simulink model "Actuator_Control"  (R2014a)
settings: Solver=FixedStepDiscrete  StartTime=0.0  StopTime=inf  FixedStep=sample_time  RelTol=1e-3
values from neighbouring files (symbols this model uses):
  A1_notch_f1 = -2*cos(fnotch_f1*sample_time)    [actuator_control_params.m]
  A2_notch_f1 = 1    [actuator_control_params.m]
  A_lpf_accel = 1 + B1_lpf_accel + B2_lpf_accel    [actuator_control_params.m]
  A_lpf_dtau = 1 + B1_lpf_dtau + B2_lpf_dtau    [actuator_control_params.m]
  B1_lpf_accel = -2*exp(-lpf_damping*fcut_acceleration*sample_time)*cos(fcut_acceleration*sample_time*sqrt(1-lpf_damping^2))    [actuator_control_params.m]
  B1_lpf_dtau = -2*exp(-lpf_damping*fcut_dtau*sample_time)*cos(fcut_dtau*sample_time*sqrt(1-lpf_damping^2))    [actuator_control_params.m]
  B1_notch_f1 = -2*exp(-notch_damping*fnotch_f1*sample_time)*cos(fnotch_f1*sample_time*sqrt(1-notch_damping^2))    [actuator_control_params.m]
  B2_lpf_accel = exp(-2*lpf_damping*fcut_acceleration*sample_time)    [actuator_control_params.m]
  B2_lpf_dtau = exp(-2*lpf_damping*fcut_dtau*sample_time)    [actuator_control_params.m]
  B2_notch_f1 = exp(-2*notch_damping*fnotch_f1*sample_time)    [actuator_control_params.m]
  j_segments = [0.145 0.155 0.145 0.155]    [model_params.m]
  k_ff = 1    [actuator_control_params.m]
  K_notch_f1 = (1+B1_notch_f1+B2_notch_f1)/(1+A1_notch_f1+A2_notch_f1)    [actuator_control_params.m]
  k_sea = [4255.0 4525.3 4372.1 4322.4]    [model_params.m]
  kd_sea_torque_flight = 0.3*sqrt(2)/2*2*sqrt(k_sea.*j_segments) ./ k_sea    [actuator_control_params.m]
  kd_sea_torque_stance = sqrt(2)/2*2*sqrt(k_sea.*(4.4)) ./ k_sea    [actuator_control_params.m]
  kp_sea_torque_flight = 0.3    [actuator_control_params.m]
  kp_sea_torque_stance = 8    [actuator_control_params.m]
  lateral_torque_ramp_time = control_start_time+2    (= 11)    [actuator_control_params.m]
  max_sagittal_loaded_torque = LEG_MTR_MAX_TORQUE    [actuator_control_params.m]
  max_sagittal_unloaded_torque = LEG_MTR_MAX_CONT_TORQUE    [actuator_control_params.m]
  sagittal_torque_ramp_time = sagittal_starting_time+5    (= 18)    [actuator_control_params.m]
  sea_control_torque_cmd_small_threshold = 1*ones(1,4)    [actuator_control_params.m]
  sea_coulomb_friction = [18.69 26.08 25.95 26.8+5]    [actuator_control_params.m]
  sea_coulomb_friction_direction_switch_sensitivity = [15 5 15 15]    [actuator_control_params.m]
  sea_extra_sliding_friction = 0.001*ones(1,4)    [actuator_control_params.m]
  sea_offset_friction = [7.659 -6.198 6.447 -6.594]    [actuator_control_params.m]
  stance_flight_torque_threshold = 40*ones(1,4)    [actuator_control_params.m]
undefined symbols (not defined in the file or in its folder): sample_time
libraries: simulink x7
settings Model: BufferReuse=off  Creator=wmartin  LastModifiedBy=wmartin
settings SolverCC: EnableConcurrentExecution=on
settings DataIOCC: SaveOutput=off  SaveTime=off
settings OptimizationCC: BlockReduction=off  OptimizeBlockIOStorage=off  BufferReuse=off  GlobalBufferReuse=off  ExpressionFolding=off  LocalBlockOutputs=off  SimCompilerOptimization=On
settings HardwareCC: ProdIntDivRoundTo=Zero  ProdEndianess=LittleEndian  ProdHWDeviceType=Generic->32-bit x86 compatible
settings ModelReferenceCC: ModelReferenceNumInstancesAllowed=Single  ModelReferenceMinAlgLoopOccurrences=on
settings RTWCC: SystemTargetFile=slrt.tlc  TemplateMakefile=slrt_default_tmf  Description=Simulink Real-Time  RTWVerbose=off  ProcessScript=slrt_make_rtw_hook  RTWCompilerOptimization=On
settings SimulinkRealTimeCC: GeneratePreprocessorConditionals=Disable all  EnableShiftOperators=on  RL32LogBufSizeModifier=100000000

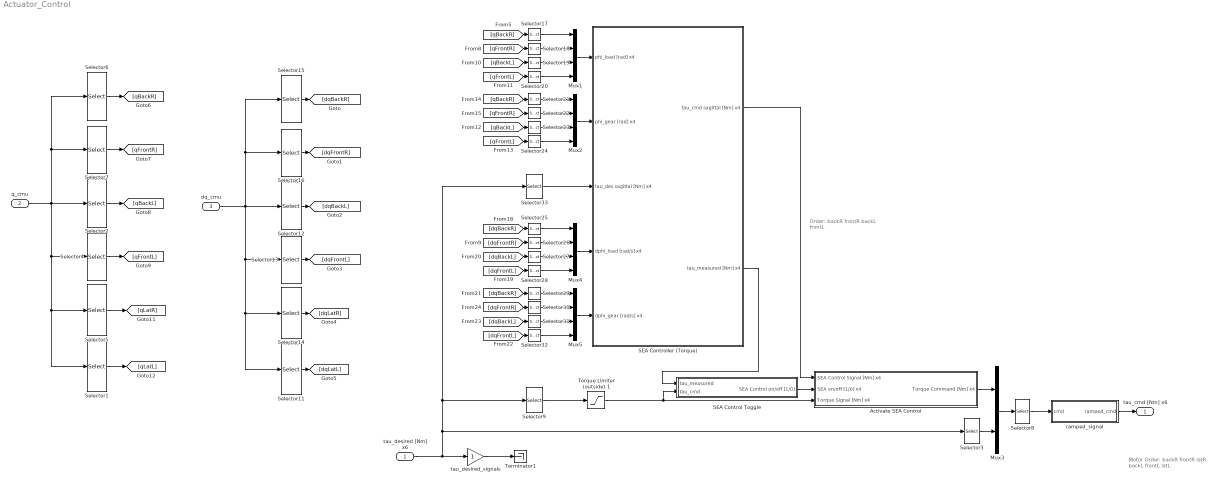
== system Actuator_Control ==
  note: Order:
      | backR
      | frontR
      | backL
      | frontL
  note: Motor Order:
      |
      | backR
      | frontR
      | latR
      | backL
      | frontL
      | latL
  tau_desired [Nm] x6 : Inport  OutDataTypeStr=double  PortDimensions=6  SampleTime=0
  q_cmu : Inport  Port=2  OutDataTypeStr=double  PortDimensions=13  SampleTime=0
  dq_cmu : Inport  Port=3  OutDataTypeStr=double  PortDimensions=13  SampleTime=0
  Activate SEA Control : Subsystem
  Mux{1..2,4..5} (4 alike) : Mux
  Mux3 : Mux  Inputs=2
  SEA Control Toggle : Subsystem
  SEA Controller (Torque) : Subsystem
  Selector1 : Selector  InputPortWidth=13  Indices=[10]
  Selector11 : Selector  InputPortWidth=13  Indices=[10]
  Selector12 : Selector  InputPortWidth=13  Indices=[5 6]
  Selector13 : Selector  InputPortWidth=13  Indices=[7 8]
  Selector14 : Selector  InputPortWidth=13  Indices=[9]
  Selector15 : Selector  InputPortWidth=13  Indices=[1 2]
  Selector16 : Selector  InputPortWidth=13  Indices=[3 4]
  Selector{17..20,25..28} (8 alike) : Selector  InputPortWidth=2  Indices=[1]
  Selector2 : Selector  InputPortWidth=13  Indices=[5 6]
  Selector{21..24,29..32} (8 alike) : Selector  InputPortWidth=2  Indices=[2]
  Selector3 : Selector  InputPortWidth=6  Indices=[3 6]
  Selector33 : Selector  InputPortWidth=6  Indices=[1 2 4 5]
  Selector4 : Selector  InputPortWidth=13  Indices=[7 8]
  Selector5 : Selector  InputPortWidth=13  Indices=[9]
  Selector6 : Selector  InputPortWidth=13  Indices=[1 2]
  Selector7 : Selector  InputPortWidth=13  Indices=[3 4]
  Selector8 : Selector  InputPortWidth=6  Indices=[1 2 5 3 4 6]
  Selector9 : Selector  InputPortWidth=6  Indices=[1 2 4 5]
  Terminator1 : Terminator
  Torque Limiter (outside) 1 : Saturate  UpperLimit=max_sagittal_unloaded_torque  LowerLimit=-max_sagittal_unloaded_torque
      settings: AttributesFormatString=Hi: %<UpperLimit>\nLo: %<LowerLimit>
  ramped_signal : Subsystem
  tau_desired_signals : Gain  Description=xPCTag(1)=tau_cmd_signal;
  tau_cmd [Nm] x6 : Outport  OutDataTypeStr=double  PortDimensions=6  SampleTime=0  InitialOutput=[0 0 0 0 0 0]
  wires:
  Selector9/1 -> Torque Limiter (outside) 1/1
  SEA Controller (Torque)/2(tau_measured [Nm] x4) -> SEA Control Toggle/1(tau_measured)
  SEA Control Toggle/1(SEA Control on/off [1/0]) -> Activate SEA Control/2("SEA on/off [1/0] x4 ")
  SEA Controller (Torque)/1(tau_cmd sagittal [Nm] x4) -> Activate SEA Control/1(SEA Control Signal [Nm] x4)
  Torque Limiter (outside) 1/1 -> Activate SEA Control/3(Torque Signal [Nm] x4), SEA Control Toggle/2(tau_cmd)
  Activate SEA Control/1(Torque Command [Nm] x4) -> Mux3/1
  tau_desired [Nm] x6/1 -> Selector33/1, Selector9/1, Selector3/1, tau_desired_signals/1
  ramped_signal/1(ramped_cmd) -> tau_cmd [Nm] x6/1
  tau_desired_signals/1 -> Terminator1/1
  Selector5/1 -> [qLatR]
  Selector1/1 -> [qLatL]
  Selector6/1 -> [qBackR]
  Selector7/1 -> [qFrontR]
  Selector2/1 -> [qBackL]
  Selector4/1 -> [qFrontL]
  q_cmu/1 -> Selector2/1, Selector7/1, Selector6/1, Selector4/1, Selector5/1, Selector1/1
  Selector8/1 -> ramped_signal/1(cmd)
  dq_cmu/1 -> Selector11/1, Selector14/1, Selector13/1, Selector15/1, Selector16/1, Selector12/1
  Selector14/1 -> [dqLatR]
  Selector11/1 -> [dqLatL]
  Selector15/1 -> [dqBackR]
  Selector16/1 -> [dqFrontR]
  Selector12/1 -> [dqBackL]
  Selector13/1 -> [dqFrontL]
  Mux1/1 -> SEA Controller (Torque)/1(phi_load [rad] x4)
  [qBackR] -> Selector17/1
  Selector17/1 -> Mux1/1
  Selector19/1 -> Mux1/3
  Selector18/1 -> Mux1/2
  Selector20/1 -> Mux1/4
  [qFrontR] -> Selector18/1
  [qBackL] -> Selector19/1
  [qFrontL] -> Selector20/1
  Mux2/1 -> SEA Controller (Torque)/2(phi_gear [rad] x4)
  [qBackR] -> Selector21/1
  Selector21/1 -> Mux2/1
  Selector23/1 -> Mux2/3
  Selector22/1 -> Mux2/2
  Selector24/1 -> Mux2/4
  [qFrontR] -> Selector22/1
  [qBackL] -> Selector23/1
  [qFrontL] -> Selector24/1
  Mux4/1 -> SEA Controller (Torque)/4(dphi_load [rad/s] x4)
  [dqBackR] -> Selector25/1
  Selector25/1 -> Mux4/1
  Selector27/1 -> Mux4/3
  Selector26/1 -> Mux4/2
  Selector28/1 -> Mux4/4
  [dqFrontR] -> Selector26/1
  [dqBackL] -> Selector27/1
  [dqFrontL] -> Selector28/1
  Mux5/1 -> SEA Controller (Torque)/5(dphi_gear [rad/s] x4)
  [dqBackR] -> Selector29/1
  Selector29/1 -> Mux5/1
  Selector31/1 -> Mux5/3
  Selector30/1 -> Mux5/2
  Selector32/1 -> Mux5/4
  [dqFrontR] -> Selector30/1
  [dqBackL] -> Selector31/1
  [dqFrontL] -> Selector32/1
  Selector33/1 -> SEA Controller (Torque)/3(tau_des sagittal [Nm] x4)
  Selector3/1 -> Mux3/2
  Mux3/1 -> Selector8/1

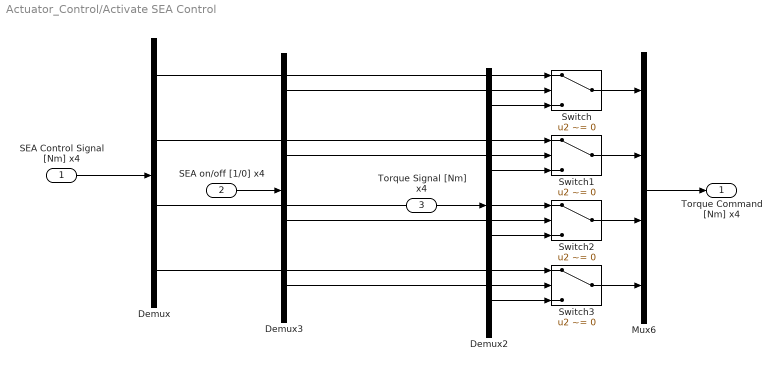
== system Actuator_Control/Activate SEA Control ==
  SEA Control Signal [Nm] x4 : Inport
  "SEA on/off [1/0] x4 " : Inport  Port=2
  Torque Signal [Nm] x4 : Inport  Port=3
  Demux : Demux
  Demux2 : Demux
  Demux3 : Demux
  Mux6 : Mux
  Switch{,1..3} (4 alike) : Switch  Criteria=u2 ~= 0
  Torque Command [Nm] x4 : Outport
  wires:
  Demux2/2 -> Switch1/3
  Demux2/1 -> Switch/3
  Demux/1 -> Switch/1
  Switch/1 -> Mux6/1
  Switch1/1 -> Mux6/2
  Switch3/1 -> Mux6/4
  Demux3/1 -> Switch/2
  Mux6/1 -> Torque Command [Nm] x4/1
  Demux3/3 -> Switch2/2
  Demux3/2 -> Switch1/2
  Demux/3 -> Switch2/1
  Switch2/1 -> Mux6/3
  Demux/4 -> Switch3/1
  Demux2/4 -> Switch3/3
  Demux3/4 -> Switch3/2
  Demux/2 -> Switch1/1
  Demux2/3 -> Switch2/3
  SEA Control Signal [Nm] x4/1 -> Demux/1
  "SEA on/off [1/0] x4 "/1 -> Demux3/1
  Torque Signal [Nm] x4/1 -> Demux2/1

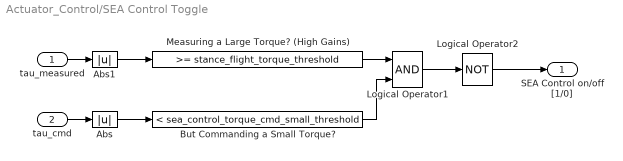
== system Actuator_Control/SEA Control Toggle ==
  tau_measured : Inport
  tau_cmd : Inport  Port=2
  Abs : Abs
  Abs1 : Abs
  But Commanding a Small Torque? : simulink/Logic and Bit Operations/Compare To Constant  relop=<  const=sea_control_torque_cmd_small_threshold  OutDataTypeStr=boolean
  Logical Operator1 : Logic  AllPortsSameDT=off  OutDataTypeStr=boolean
  Logical Operator2 : Logic  Operator=NOT  AllPortsSameDT=off  OutDataTypeStr=boolean
  Measuring a Large Torque? (High Gains) : simulink/Logic and Bit Operations/Compare To Constant  relop=>=  const=stance_flight_torque_threshold  OutDataTypeStr=boolean
  SEA Control on/off [1/0] : Outport
  wires:
  Logical Operator2/1 -> SEA Control on/off [1/0]/1
  But Commanding a Small Torque?/1 -> Logical Operator1/2
  Logical Operator1/1 -> Logical Operator2/1
  tau_cmd/1 -> Abs/1
  Abs/1 -> But Commanding a Small Torque?/1
  tau_measured/1 -> Abs1/1
  Measuring a Large Torque? (High Gains)/1 -> Logical Operator1/1
  Abs1/1 -> Measuring a Large Torque? (High Gains)/1

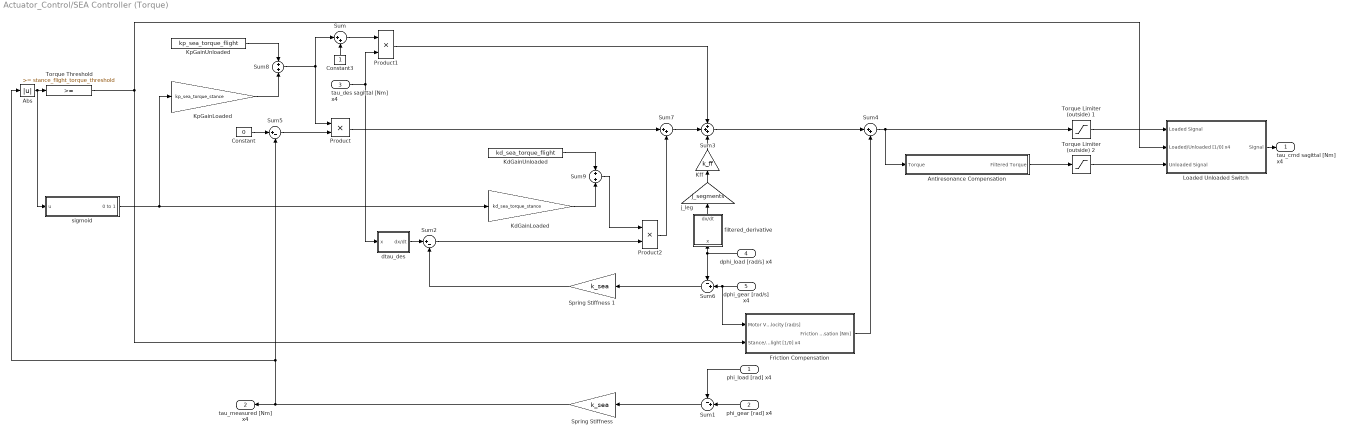
== system Actuator_Control/SEA Controller (Torque) ==
  phi_load [rad] x4 : Inport
  phi_gear [rad] x4 : Inport  Port=2
  tau_des sagittal [Nm] x4 : Inport  Port=3
  dphi_load [rad/s] x4 : Inport  Port=4
  dphi_gear [rad/s] x4 : Inport  Port=5
  Abs : Abs
  Antiresonance Compensation : Subsystem
  Constant : Constant  Value=0
  Constant3 : Constant
  Friction Compensation : Subsystem
  KdGainLoaded : Gain  Description=xPCTag(1)=kd_sea_torque;  Gain=kd_sea_torque_stance
  KdGainUnloaded : Constant  Value=kd_sea_torque_flight  SampleTime=sample_time
  Kff : Gain  Gain=k_ff
  KpGainLoaded : Gain  Description=xPCTag(1)=kd_sea_torque;  Gain=kp_sea_torque_stance
  KpGainUnloaded : Constant  Value=kp_sea_torque_flight  SampleTime=sample_time
  Loaded Unloaded Switch : Subsystem
  Product : Product  SampleTime=sample_time  RndMeth=Zero
  Product1 : Product  RndMeth=Zero
  Product2 : Product  RndMeth=Zero
  Spring Stiffness : Gain  Gain=k_sea
  Spring Stiffness 1 : Gain  Gain=k_sea
  Sum : Sum  Inputs=|++  SampleTime=sample_time
  Sum1 : Sum  Inputs=-+|
  Sum2 : Sum  Inputs=|+-
  Sum3 : Sum  Inputs=+++
  Sum4 : Sum  Inputs=|++
  Sum5 : Sum  Inputs=|+-
  Sum6 : Sum  Inputs=-+|
  Sum7 : Sum  Inputs=|++
  Sum8 : Sum  Inputs=+|+  SampleTime=sample_time
  Sum9 : Sum  Inputs=+|+  SampleTime=sample_time
  Torque Limiter (outside) 1 : Saturate  UpperLimit=max_sagittal_loaded_torque  LowerLimit=-max_sagittal_loaded_torque
      settings: AttributesFormatString=Hi: %<UpperLimit>\nLo: %<LowerLimit>
  Torque Limiter (outside) 2 : Saturate  UpperLimit=max_sagittal_unloaded_torque  LowerLimit=-max_sagittal_unloaded_torque
      settings: AttributesFormatString=Hi: %<UpperLimit>\nLo: %<LowerLimit>
  Torque Threshold : simulink/Logic and Bit Operations/Compare To Constant  relop=>=  const=stance_flight_torque_threshold  OutDataTypeStr=boolean
  dtau_des : Subsystem
  filtered_derivative : Subsystem
  j_leg : Gain  Description=xPCTag(1)=kd_sea_torque;  Gain=j_segments
  sigmoid : Subsystem
  tau_cmd sagittal [Nm] x4 : Outport
  tau_measured [Nm] x4 : Outport  Port=2
  wires:
  Antiresonance Compensation/1(Filtered Torque) -> Torque Limiter (outside) 2/1
  Sum3/1 -> Sum4/1
  Sum7/1 -> Sum3/2
  Product1/1 -> Sum3/1
  Sum4/1 -> Antiresonance Compensation/1(Torque), Torque Limiter (outside) 1/1
  Abs/1 -> sigmoid/1(u), Torque Threshold/1
  Sum8/1 -> Sum/1, Product/1
  Spring Stiffness/1 -> tau_measured [Nm] x4/1, Abs/1, Sum5/2
  Torque Threshold/1 -> Loaded Unloaded Switch/2(Loaded/Unloaded [1/0] x4), Friction Compensation/2(Stance/Flight [1/0] x4)
  Sum1/1 -> Spring Stiffness/1
  phi_load [rad] x4/1 -> Sum1/1
  phi_gear [rad] x4/1 -> Sum1/2
  Constant/1 -> Sum5/1
  dtau_des/1(dx/dt) -> Sum2/1
  Sum6/1 -> Spring Stiffness 1/1
  Spring Stiffness 1/1 -> Sum2/2
  dphi_load [rad/s] x4/1 -> Sum6/1, filtered_derivative/1(x)
  dphi_gear [rad/s] x4/1 -> Friction Compensation/1(Motor Velocity [rad/s]), Sum6/2
  Sum5/1 -> Product/2
  Product/1 -> Sum7/1
  Constant3/1 -> Sum/2
  Sum/1 -> Product1/1
  filtered_derivative/1(dx/dt) -> j_leg/1
  j_leg/1 -> Kff/1
  Torque Limiter (outside) 1/1 -> Loaded Unloaded Switch/1(Loaded Signal)
  Kff/1 -> Sum3/3
  tau_des sagittal [Nm] x4/1 -> dtau_des/1(x), Product1/2
  Friction Compensation/1(Friction Compensation [Nm]) -> Sum4/2
  Torque Limiter (outside) 2/1 -> Loaded Unloaded Switch/3(Unloaded Signal)
  Loaded Unloaded Switch/1(Signal) -> tau_cmd sagittal [Nm] x4/1
  KpGainUnloaded/1 -> Sum8/1
  KpGainLoaded/1 -> Sum8/2
  KdGainUnloaded/1 -> Sum9/1
  KdGainLoaded/1 -> Sum9/2
  sigmoid/1(0 to 1) -> KpGainLoaded/1, KdGainLoaded/1
  Sum2/1 -> Product2/2
  Sum9/1 -> Product2/1
  Product2/1 -> Sum7/2

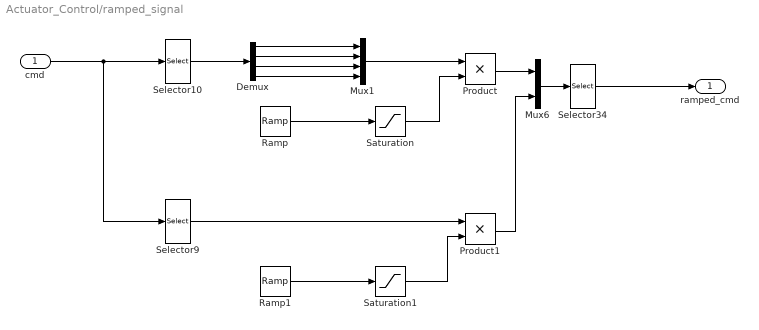
== system Actuator_Control/ramped_signal ==
  cmd : Inport
  Demux : Demux
  Mux1 : Mux
  Mux6 : Mux  Inputs=2
  Product : Product  RndMeth=Zero
  Product1 : Product  RndMeth=Zero
  Ramp : simulink/Sources/Ramp  slope=1/sagittal_torque_ramp_time  start=sagittal_starting_time  X0=0
      settings: AttributesFormatString=Start: %<start>\nSlope: %<slope>
  Ramp1 : simulink/Sources/Ramp  slope=1/lateral_torque_ramp_time  start=control_start_time  X0=0
      settings: AttributesFormatString=Start: %<start>\nSlope: %<slope>
  Saturation : Saturate  UpperLimit=1  LowerLimit=0
      settings: AttributesFormatString=Hi: %<UpperLimit>\nLo: %<LowerLimit>
  Saturation1 : Saturate  UpperLimit=1  LowerLimit=0
      settings: AttributesFormatString=Hi: %<UpperLimit>\nLo: %<LowerLimit>
  Selector10 : Selector  InputPortWidth=6  Indices=[1 2 4 5]
  Selector34 : Selector  InputPortWidth=6  Indices=[1 2 5 3 4 6]
  Selector9 : Selector  InputPortWidth=6  Indices=[3 6]
  ramped_cmd : Outport
  wires:
  Selector9/1 -> Product1/1
  Saturation1/1 -> Product1/2
  Ramp1/1 -> Saturation1/1
  Saturation/1 -> Product/2
  Ramp/1 -> Saturation/1
  Product/1 -> Mux6/1
  cmd/1 -> Selector10/1, Selector9/1
  Product1/1 -> Mux6/2
  Selector34/1 -> ramped_cmd/1
  Selector10/1 -> Demux/1
  Mux6/1 -> Selector34/1
  Demux/1 -> Mux1/1
  Demux/2 -> Mux1/2
  Mux1/1 -> Product/1
  Demux/4 -> Mux1/4
  Demux/3 -> Mux1/3

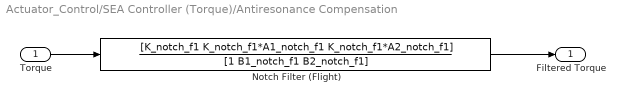
== system Actuator_Control/SEA Controller (Torque)/Antiresonance Compensation ==
  Torque : Inport
  Notch Filter (Flight) : DiscreteTransferFcn  Numerator=[K_notch_f1 K_notch_f1*A1_notch_f1 K_notch_f1*A2_notch_f1]  Denominator=[1 B1_notch_f1 B2_notch_f1]  SampleTime=sample_time
  Filtered Torque : Outport
  wires:
  Torque/1 -> Notch Filter (Flight)/1
  Notch Filter (Flight)/1 -> Filtered Torque/1

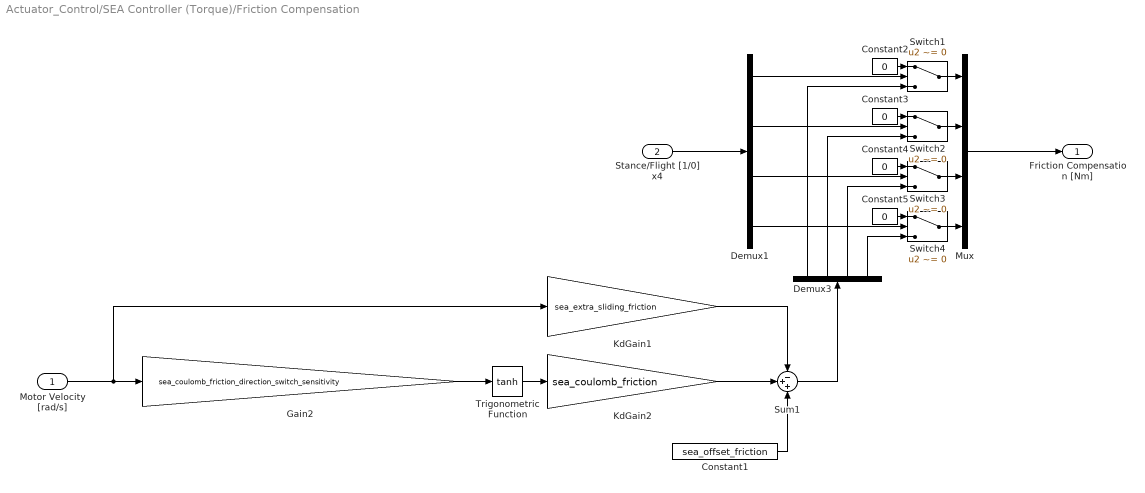
== system Actuator_Control/SEA Controller (Torque)/Friction Compensation ==
  Motor Velocity [rad/s] : Inport
  Stance/Flight [1/0] x4 : Inport  Port=2
  Constant1 : Constant  Value=sea_offset_friction
  Constant{2..5} (4 alike) : Constant  Value=0
  Demux1 : Demux
  Demux3 : Demux
  Gain2 : Gain  Gain=sea_coulomb_friction_direction_switch_sensitivity
  KdGain1 : Gain  Description=xPCTag(1)=kd_sea_torque;  Gain=sea_extra_sliding_friction
  KdGain2 : Gain  Description=xPCTag(1)=kd_sea_torque;  Gain=sea_coulomb_friction
  Mux : Mux
  Sum1 : Sum  Inputs=-++
  Switch{1..4} (4 alike) : Switch  Criteria=u2 ~= 0
  Trigonometric Function : Trigonometry  Operator=tanh
  Friction Compensation [Nm] : Outport
  wires:
  Sum1/1 -> Demux3/1
  Constant5/1 -> Switch4/1
  Constant4/1 -> Switch3/1
  Constant3/1 -> Switch2/1
  Constant2/1 -> Switch1/1
  Stance/Flight [1/0] x4/1 -> Demux1/1
  Demux3/1 -> Switch1/3
  Demux3/2 -> Switch2/3
  Demux3/3 -> Switch3/3
  Demux3/4 -> Switch4/3
  Demux1/1 -> Switch1/2
  Switch1/1 -> Mux/1
  Switch4/1 -> Mux/4
  Switch3/1 -> Mux/3
  Switch2/1 -> Mux/2
  Demux1/2 -> Switch2/2
  Demux1/3 -> Switch3/2
  Demux1/4 -> Switch4/2
  Constant1/1 -> Sum1/3
  KdGain2/1 -> Sum1/2
  Motor Velocity [rad/s]/1 -> KdGain1/1, Gain2/1
  Gain2/1 -> Trigonometric Function/1
  Trigonometric Function/1 -> KdGain2/1
  Mux/1 -> Friction Compensation [Nm]/1
  KdGain1/1 -> Sum1/1

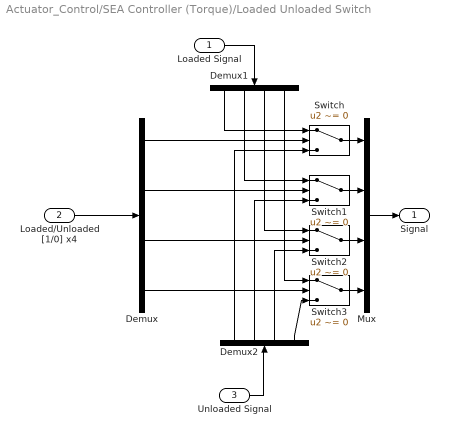
== system Actuator_Control/SEA Controller (Torque)/Loaded Unloaded Switch ==
  Loaded Signal : Inport
  Loaded/Unloaded [1/0] x4 : Inport  Port=2
  Unloaded Signal : Inport  Port=3
  Demux : Demux
  Demux1 : Demux
  Demux2 : Demux
  Mux : Mux
  Switch{,1..3} (4 alike) : Switch  Criteria=u2 ~= 0
  Signal : Outport
  wires:
  Demux/4 -> Switch3/2
  Demux/3 -> Switch2/2
  Demux/2 -> Switch1/2
  Switch1/1 -> Mux/2
  Switch2/1 -> Mux/3
  Switch3/1 -> Mux/4
  Loaded/Unloaded [1/0] x4/1 -> Demux/1
  Mux/1 -> Signal/1
  Switch/1 -> Mux/1
  Demux/1 -> Switch/2
  Loaded Signal/1 -> Demux1/1
  Demux1/1 -> Switch/1
  Demux1/2 -> Switch1/1
  Demux1/3 -> Switch2/1
  Demux1/4 -> Switch3/1
  Unloaded Signal/1 -> Demux2/1
  Demux2/4 -> Switch3/3
  Demux2/3 -> Switch2/3
  Demux2/2 -> Switch1/3
  Demux2/1 -> Switch/3

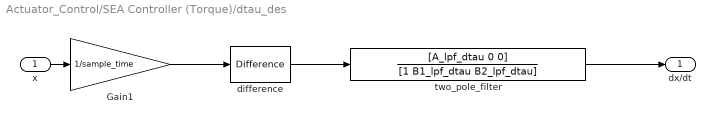
== system Actuator_Control/SEA Controller (Torque)/dtau_des ==
  x : Inport
  Gain1 : Gain  Gain=1/sample_time
  difference : simulink/Discrete/Difference  ICPrevInput=0.0  InputProcessing=Inherited  OutMin=[]  OutMax=[]  OutDataType=fixdt(1, 16)  OutScaling=2^-10  DoSatur=off
  two_pole_filter : DiscreteTransferFcn  Numerator=[A_lpf_dtau 0 0]  Denominator=[1 B1_lpf_dtau B2_lpf_dtau]  SampleTime=sample_time
  dx/dt : Outport
  wires:
  Gain1/1 -> difference/1
  difference/1 -> two_pole_filter/1
  x/1 -> Gain1/1
  two_pole_filter/1 -> dx/dt/1

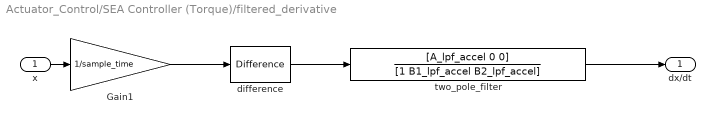
== system Actuator_Control/SEA Controller (Torque)/filtered_derivative ==
  x : Inport
  Gain1 : Gain  Gain=1/sample_time
  difference : simulink/Discrete/Difference  ICPrevInput=0.0  InputProcessing=Inherited  OutMin=[]  OutMax=[]  OutDataType=fixdt(1, 16)  OutScaling=2^-10  DoSatur=off
  two_pole_filter : DiscreteTransferFcn  Numerator=[A_lpf_accel 0 0]  Denominator=[1 B1_lpf_accel B2_lpf_accel]  SampleTime=sample_time
  dx/dt : Outport
  wires:
  two_pole_filter/1 -> dx/dt/1
  x/1 -> Gain1/1
  difference/1 -> two_pole_filter/1
  Gain1/1 -> difference/1

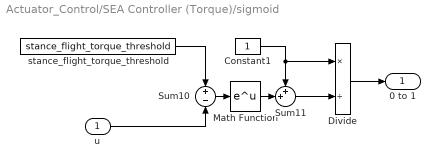
== system Actuator_Control/SEA Controller (Torque)/sigmoid ==
  u : Inport
  Constant1 : Constant
  Divide : Product  Inputs=*/
  Math Function : Math  SaturateOnIntegerOverflow=on
  Sum10 : Sum  Inputs=+|-  SampleTime=sample_time
  Sum11 : Sum  Inputs=++|  SampleTime=sample_time
  stance_flight_torque_threshold : Constant  Value=stance_flight_torque_threshold  SampleTime=sample_time
  0 to 1 : Outport
  wires:
  Divide/1 -> 0 to 1/1
  Sum10/1 -> Math Function/1
  stance_flight_torque_threshold/1 -> Sum10/1
  Constant1/1 -> Sum11/1, Divide/1
  Math Function/1 -> Sum11/2
  u/1 -> Sum10/2
  Sum11/1 -> Divide/2
